simulink model "SpringMassDamper"  (R2015a)
settings: Solver=ode45  StartTime=0.0  StopTime=10.0  RelTol=1e-3
undefined symbols (not defined in the file): sigbuilder_block
libraries: fl_lib x12, nesl_utility x4
settings Model: Creator=nightstalker  LastModifiedBy=nightstalker

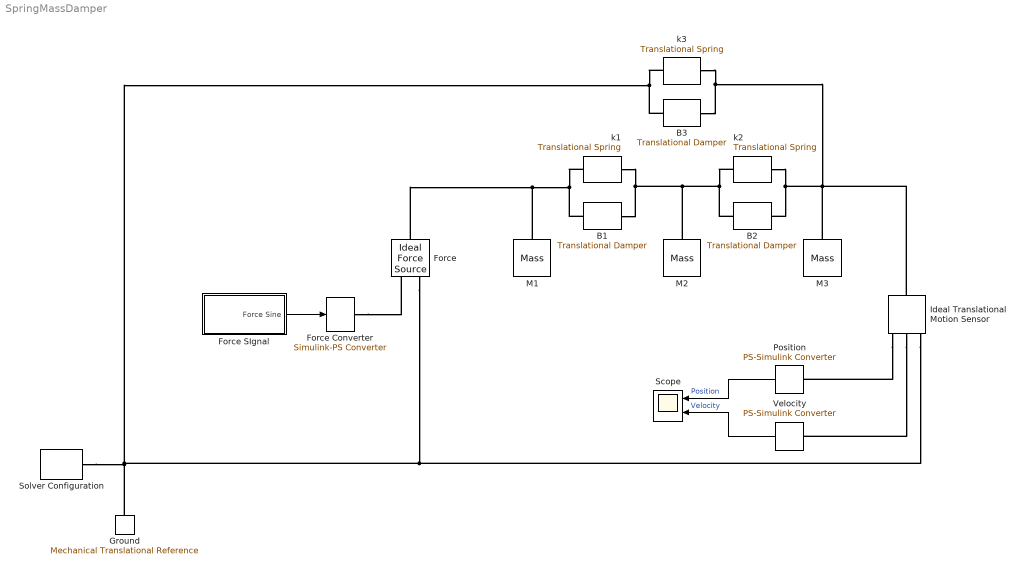
== system SpringMassDamper ==
  B1 : fl_lib/Mechanical/Translational Elements/Translational Damper  D=.1 N/(m/s)  v_specify=off  v_priority=High  v=0 m/s  f_specify=off  f_priority=High  f=0 N
  B2 : fl_lib/Mechanical/Translational Elements/Translational Damper  D=10 N/(m/s)  v_specify=off  v_priority=High  v=0 m/s  f_specify=off  f_priority=High  f=0 N
  B3 : fl_lib/Mechanical/Translational Elements/Translational Damper  D=10 N/(m/s)  v_specify=off  v_priority=High  v=0 m/s  f_specify=off  f_priority=High  f=0 N
  Force : fl_lib/Mechanical/Mechanical Sources/Ideal Force Source
  Force Converter : nesl_utility/Simulink-PS Converter  PhysicalDomain=network_engine_domain  SubClassName=ps_input  LeftPortType=input  RightPortType=output  PseudoPeriodic=off  Frequencies=[]  NoiseDistribution=none  NoiseParameters=[]  Unit=1  AffineConversion=off  InputFiltering=off  SimscapeFilterOrder=1  InputFilterTimeConstant=0.001  UdotUserProvided=1
  Force SIgnal : Subsystem  Tag=STV Subsys  LoadFcn=sigbuilder_block('load');  StartFcn=sigbuilder_block('start');  StopFcn=sigbuilder_block('stop');  ClipboardFcn=sigbuilder_block('clipboard');  mask(Sigbuilder block){}
      mask help: Simulink:masks:SigbuilderBlock_MD
      mask init:
      | if ~strcmp(get_param(bdroot(gcbh),'SimulationStatus'),'stopped') tuvar = sigbuilder_block('maskInit'); end
      settings: CopyFcn=sigbuilder_block('copy');  DeleteFcn=sigbuilder_block('delete');  ModelCloseFcn=sigbuilder_block('modelClose');  PreSaveFcn=sigbuilder_block('preSave');  PauseFcn=sigbuilder_block('pause');  ContinueFcn=sigbuilder_block('continue');  NameChangeFcn=sigbuilder_block('namechange');  OpenFcn=sigbuilder_block('open',[437.6 199.2 550.4 400 ]);  CloseFcn=sigbuilder_block('close');
      mask Display: plot(0, 0, 100, 100,[2, 2, 32, 32, 2], [68, 8, 8, 68, 68],[32, 2], [38, 38], [32, 19, 2],[53, 60, 44], [32, 17, 17, 2],[16, 16, 31, 31]);txt = getActiveGroup(gcbh);text(2, 100, txt,'verticalAlignment', 'top');
  Ground : fl_lib/Mechanical/Translational Elements/Mechanical Translational Reference
  Ideal Translational Motion Sensor : fl_lib/Mechanical/Mechanical Sensors/Ideal Translational Motion Sensor  offset=0 m
  M1 : fl_lib/Mechanical/Translational Elements/Mass  mass=1 kg  v_specify=off  v_priority=High  v=0 m/s  f_specify=off  f_priority=High  f=0 N
  M2 : fl_lib/Mechanical/Translational Elements/Mass  mass=1 kg  v_specify=off  v_priority=High  v=0 m/s  f_specify=off  f_priority=High  f=0 N
  M3 : fl_lib/Mechanical/Translational Elements/Mass  mass=1 kg  v_specify=off  v_priority=High  v=0 m/s  f_specify=off  f_priority=High  f=0 N
  Position : nesl_utility/PS-Simulink Converter  PhysicalDomain=network_engine_domain  SubClassName=ps_output  LeftPortType=input  RightPortType=output  PseudoPeriodic=off  Frequencies=[]  Unit=1  AffineConversion=off
  Scope : Scope  NumInputPorts=2
      settings: YMin=-5~-5  YMax=5~5
  Solver Configuration : nesl_utility/Solver Configuration  PhysicalDomain=network_engine_domain  SubClassName=solver  LeftPortType=input  RightPortType=generic  Accelerate=off  Tones=[]  Harmonics=[]  SimulateNoise=off  Profile=off  UseLocalSampling=off  EnableSwitchedLinearOptims=on  FrequencyDomain=off  UseCCode=off  RelTol=0.001  AbsTol=1e-06  MinStep=1e-09  ToWorkspace=off  RevertToSquareIcSolve=off  NumHomotopyIterations=100  DoDC=off  ResidualTolerance=1e-09  UseLocalSolver=off  LocalSolverChoice=NE_BACKWARD_EULER_ADVANCER  LocalSolverSampleTime=0.001  DoFixedCost=off  MaxNonlinIter=3  MaxModeIter=2  LinearAlgebra=Sparse  DelaysMemoryBudget=1024  AutomaticFiltering=on  FilteringTimeConstant=0.001
  Velocity : nesl_utility/PS-Simulink Converter  PhysicalDomain=network_engine_domain  SubClassName=ps_output  LeftPortType=input  RightPortType=output  PseudoPeriodic=off  Frequencies=[]  Unit=1  AffineConversion=off
  k1 : fl_lib/Mechanical/Translational Elements/Translational Spring  spr_rate=10 N/m  v_specify=off  v_priority=High  v=0 m/s  f_specify=off  f_priority=High  f=0 N  x_specify=off  x_priority=High  x=0 m
  k2 : fl_lib/Mechanical/Translational Elements/Translational Spring  spr_rate=100 N/m  v_specify=off  v_priority=High  v=0 m/s  f_specify=off  f_priority=High  f=0 N  x_specify=off  x_priority=High  x=0 m
  k3 : fl_lib/Mechanical/Translational Elements/Translational Spring  spr_rate=100 N/m  v_specify=off  v_priority=High  v=0 m/s  f_specify=off  f_priority=High  f=0 N  x_specify=off  x_priority=High  x=0 m
  wires:
  Force SIgnal/1(Force Sine) -> Force Converter/1
  Position/1 -> Scope/1  "Position"
  Velocity/1 -> Scope/2  "Velocity"
  connections:
  M1/LConn1 -- Force/LConn1 -- B1/LConn1 -- k1/LConn1
  M2/LConn1 -- k2/LConn1 -- B2/LConn1 -- B1/RConn1 -- k1/RConn1
  B2/RConn1 -- k2/RConn1 -- M3/LConn1 -- Ideal Translational Motion Sensor/LConn1 -- B3/RConn1 -- k3/RConn1
  Ground/LConn1 -- B3/LConn1 -- k3/LConn1 -- Force/RConn2 -- Ideal Translational Motion Sensor/RConn1 -- Solver Configuration/RConn1
  Force Converter/RConn1 -- Force/RConn1
  Ideal Translational Motion Sensor/RConn3 -- Position/LConn1
  Ideal Translational Motion Sensor/RConn2 -- Velocity/LConn1

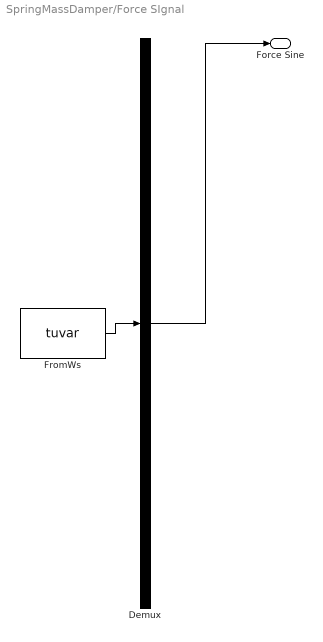
== system SpringMassDamper/Force SIgnal ==
  Demux : Demux  Tag=STV Demux  Outputs=1
  FromWs : FromWorkspace  Tag=STV FromWs  VariableName=tuvar  SampleTime=0
      SigBuilderData=|
      | common.afterFinalStr = 'Extrapolate'
      | common.sampleTime = 0
      | dataSet.timeRange = [0 10]
      | dataSet.name = 'Group 1'
      | sbobj.Groups.Name = 'Group 1'
      | sbobj.Groups.Signals.Name = 'Force Sine'
      | sbobj.Groups.Signals.XData = [0 0.0785398163397 0.157079632679 0.235619449019 0.314159265359 0.392699081699 0.471238898038 0.549778714378 0.628318530718 0.706858347058 0.785398163397 0.863937979737 0.942477796077 1.02101761242 1.09955742876 1.1780972451 1.25663706144 1.33517687778 1.41371669412 1.49225651046 1.57079632679 1.64933614313 1.72787595947 1.80641577581 1.88495559215 1.96349540849 2.04203522483 2.12057504117 2.19911485751 2.27765467385 2.35619449019 2.43473430653 2.51327412287 2.59181393921 2.67035375555 2.74889357189 2.82743338823 2.90597320457 2.98451302091 3.06305283725 3.14159265359 3.22013246993 3.29867228627 3.37721210261 3.45575191895 3.53429173529 3.61283155163 3.69137136797 3.76991118431 3.84845100065 3.92699081699 4.00553063333 4.08407044967 4.16261026601 4.24115008235 4.31968989869 4.39822971503 4.47676953137 4.55530934771 4.63384916404 4.71238898038 4.79092879672 4.86946861306 4.9480084294 5.02654824574 5.10508806208 5.18362787842 5.26216769476 5.3407075111 5.41924732744 5.49778714378 5.57632696012 5.65486677646 5.7334065928 5.81194640914 5.89048622548 5.96902604182 6.04756585816 6.1261056745 6.20464549084 6.28318530718 6.36172512352 6.44026493986 6.5188047562 6.59734457254 6.67588438888 6.75442420522 6.83296402156 6.9115038379 6.99004365424 7.06858347058 7.14712328692 7.22566310326 7.3042029196 7.38274273594 7.46128255228 7.53982236862 7.61836218496 7.69690200129 7.77544181763 7.85398163397 7.93252145031 8.01106126665 8.08960108299 8.16814089933 8.24668071567 8.32522053201 8.40376034835 8.48230016469 8.56083998103 8.63937979737 8.71791961371 8.79645943005 8.87499924639 8.95353906273 9.03207887907 9.11061869541 9.18915851175 9.26769832809 9.34623814443 9.42477796077 9.50331777711 9.58185759345 9.66039740979 9.73893722613 9.81747704247 9.89601685881 9.97455667515 10]
      | sbobj.Groups.Signals.YData = [1 8.07106781187 11 8.07106781187 1 -6.07106781187 -9 -6.07106781187 1 8.07106781187 11 8.07106781187 1 -6.07106781187 -9 -6.07106781187 1 8.07106781187 11 8.07106781187 1 -6.07106781187 -9 -6.07106781187 1 8.07106781187 11 8.07106781187 1 -6.07106781187 -9 -6.07106781187 1 8.07106781187 11 8.07106781187 1 -6.07106781187 -9 -6.07106781187 1 8.07106781187 11 8.07106781187 1 -6.07106781187 -9 -6.07106781187 1 8.07106781187 11 8.07106781187 1 -6.07106781187 -9 -6.07106781187 1 8.07106781187 11 8.07106781187 1 -6.07106781187 -9 -6.07106781187 1 8.07106781187 11 8.07106781187 1 -6.07106781187 -9 -6.07106781187 1 8.07106781187 11 8.07106781187 1 -6.07106781187 -9 -6.07106781187 1 8.07106781187 11 8.07106781187 1 -6.07106781187 -9 -6.07106781187 1 8.07106781187 11 8.07106781187 1 -6.07106781187 -9 -6.07106781187 1 8.07106781187 11 8.07106781187 1 -6.07106781187 -9 -6.07106781187 1 8.07106781187 11 8.07106781187 1 -6.07106781187 -9 -6.07106781187 1 8.07106781187 11 8.07106781187 1 -6.07106781187 -9 -6.07106781187 1 8.07106781187 11 8.07106781187 1 -6.07106781187 -9 -6.07106781187 -4.0636564111]
  Force Sine : Outport  Tag=STV Outport
  wires:
  Demux/1 -> Force Sine/1
  FromWs/1 -> Demux/1
